simulink model "test_aer_sf"  (R2012b)
settings: Solver=FixedStepDiscrete  StartTime=0.0  StopTime=0  FixedStep=0.005  RelTol=1e-3
libraries: simulink_extras x7
settings Model: Creator=HSidaoui  LastModifiedBy=HSidaoui

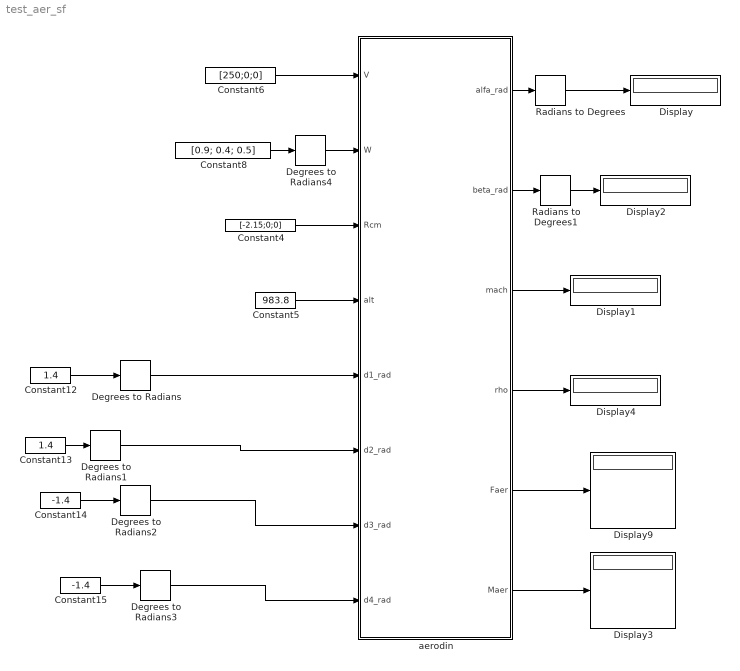
== system test_aer_sf ==
  Constant12 : Constant  Value=1.4
  Constant13 : Constant  Value=1.4
  Constant14 : Constant  Value=-1.4
  Constant15 : Constant  Value=-1.4
  Constant4 : Constant  Value=[-2.15;0;0]
  Constant5 : Constant  Value=983.8
  Constant6 : Constant  Value=[250;0;0]
  Constant8 : Constant  Value=[0.9; 0.4; 0.5]
  Degrees to Radians{,1..4} (5 alike) : simulink_extras/Transformations/Degrees to Radians
  Display{,1..4,9} (6 alike) : Display
  Radians to Degrees : simulink_extras/Transformations/Radians to Degrees
  Radians to Degrees1 : simulink_extras/Transformations/Radians to Degrees
  aerodin : Subsystem  TreatAsAtomicUnit=on
  wires:
  aerodin/1(alfa_rad) -> Radians to Degrees/1
  aerodin/3(mach) -> Display1/1
  aerodin/2(beta_rad) -> Radians to Degrees1/1
  Constant8/1 -> Degrees to Radians4/1
  Constant12/1 -> Degrees to Radians/1
  Constant13/1 -> Degrees to Radians1/1
  Constant14/1 -> Degrees to Radians2/1
  Constant15/1 -> Degrees to Radians3/1
  Radians to Degrees/1 -> Display/1
  Radians to Degrees1/1 -> Display2/1
  aerodin/6(Maer) -> Display3/1
  Constant6/1 -> aerodin/1(V)
  aerodin/5(Faer) -> Display9/1
  Degrees to Radians/1 -> aerodin/5(d1_rad)
  Degrees to Radians1/1 -> aerodin/6(d2_rad)
  Degrees to Radians2/1 -> aerodin/7(d3_rad)
  Degrees to Radians3/1 -> aerodin/8(d4_rad)
  Degrees to Radians4/1 -> aerodin/2(W)
  Constant4/1 -> aerodin/3(Rcm)
  Constant5/1 -> aerodin/4(alt)
  aerodin/4(rho) -> Display4/1

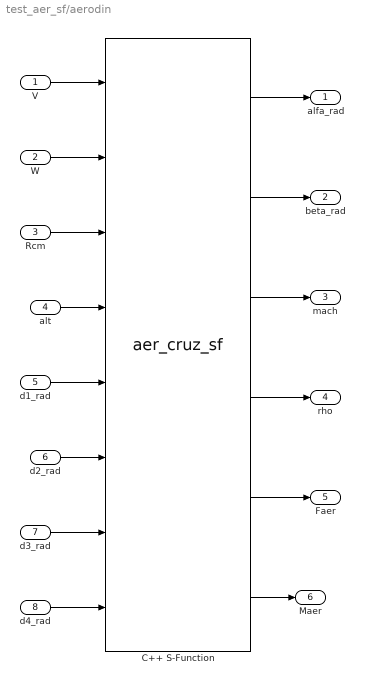
== system test_aer_sf/aerodin ==
  V : Inport
  W : Inport  Port=2
  Rcm : Inport  Port=3
  alt : Inport  Port=4
  d1_rad : Inport  Port=5
  d2_rad : Inport  Port=6
  d3_rad : Inport  Port=7
  d4_rad : Inport  Port=8
  C++ S-Function : S-Function  FunctionName=aer_cruz_sf  EnableBusSupport=off
  alfa_rad : Outport
  beta_rad : Outport  Port=2
  mach : Outport  Port=3
  rho : Outport  Port=4
  Faer : Outport  Port=5
  Maer : Outport  Port=6
  wires:
  C++ S-Function/1 -> alfa_rad/1
  C++ S-Function/2 -> beta_rad/1
  C++ S-Function/3 -> mach/1
  V/1 -> C++ S-Function/1
  W/1 -> C++ S-Function/2
  Rcm/1 -> C++ S-Function/3
  alt/1 -> C++ S-Function/4
  d1_rad/1 -> C++ S-Function/5
  d2_rad/1 -> C++ S-Function/6
  d3_rad/1 -> C++ S-Function/7
  d4_rad/1 -> C++ S-Function/8
  C++ S-Function/4 -> rho/1
  C++ S-Function/5 -> Faer/1
  C++ S-Function/6 -> Maer/1
